simulink model "inpguitest"  (Simulink 10.0)
settings: Solver=FixedStepDiscrete  StartTime=0.0  StopTime=inf  RelTol=1e-3  EnableMultiTasking=on
settings Model: Creator=nskandan  LastModifiedBy=unknown
settings DataIOCC: LimitDataPoints=on  SignalLoggingSaveFormat=ModelDataLogs
settings OptimizationCC: InitFltsAndDblsToZero=on
settings DebuggingCC: SaveWithParameterizedLinksMsg=none  SignalResolutionControl=TryResolveAllWithWarning  SolverPrmCheckMsg=warning  FcnCallInpInsideContextMsg=warning
settings SFSimCC: SimUseLocalCustomCode=on  CustomCodeUndefinedFunction=FilterOut
settings RTWCC: RTWUseLocalCustomCode=on
settings GRTTargetCC: TargetFcnLib=ansi_tfl_tmw.mat

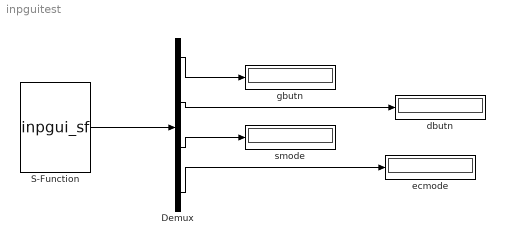
== system inpguitest ==
  Demux : Demux
  S-Function : S-Function  FunctionName=inpgui_sf  Parameters=0.005  SFunctionDeploymentMode=off  EnableBusSupport=off
  dbutn : Display
  ecmode : Display
  gbutn : Display
  smode : Display
  wires:
  S-Function/1 -> Demux/1
  Demux/1 -> gbutn/1
  Demux/2 -> dbutn/1
  Demux/3 -> smode/1
  Demux/4 -> ecmode/1
